simulink model "rotary_pendulum"  (R2022a)
settings: Solver=VariableStepAuto  StartTime=0.0  StopTime=2.5  RelTol=1e-3
values from neighbouring files (symbols this model uses):
  A = [0 0 1 0 ... (first row only)    [main.m]
  A_CL = A-B*K    [main.m]
  B = [0 ... (first row only)    [main.m]
  C = [1 0 0 0 ... (first row only)    [main.m]
  D = [0 ... (first row only)    [main.m]
  K = lqr(sys_ss, Q, R)    [main.m]
settings Model: Creator=punk  LastModifiedBy=punk

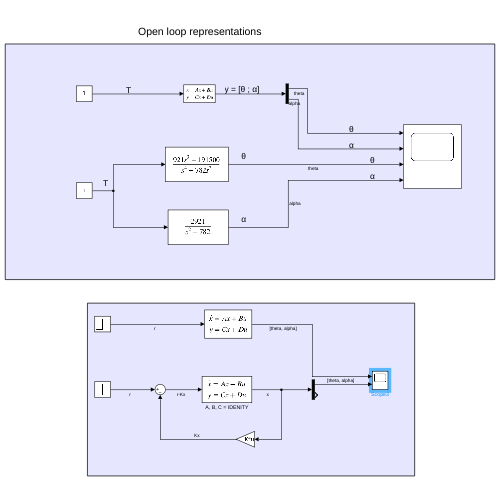
[thumbnail: Simulink's stored preview of the top-level diagram]
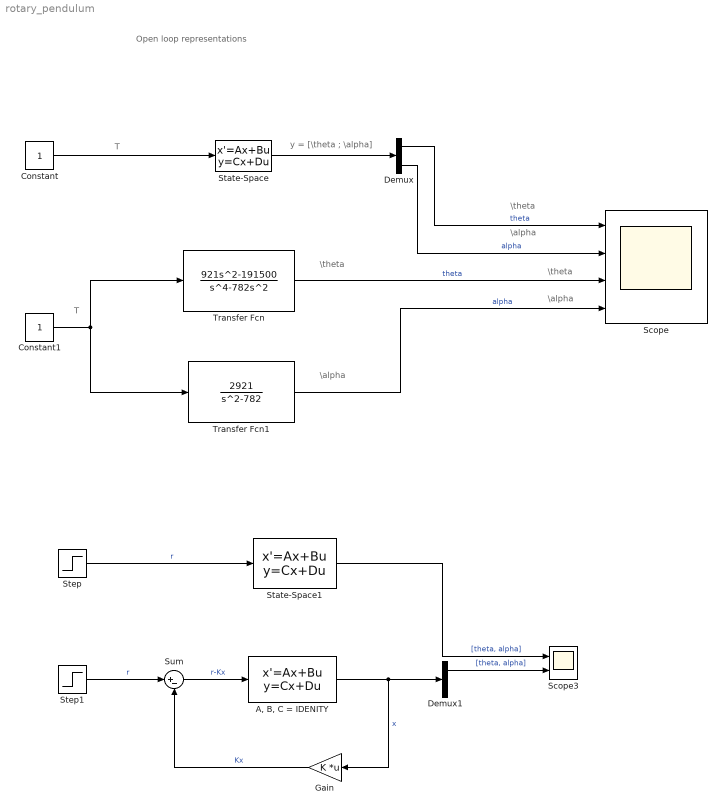
== system rotary_pendulum ==
  note: y = [\theta ; \alpha]
  note: T
  note: \alpha
  note: \theta
  note: Open loop representations
  note: T
  note: \theta
  note: \alpha
  note: \theta
  note: \alpha
  "A, B, C = IDENITY" : StateSpace  A=A  B=B  C=eye(4)  D=[0;0;0;0]  InitialCondition=0
  Constant : Constant
  Constant1 : Constant
  Demux : Demux  Outputs=2
  Demux1 : Demux  Outputs=2
  Gain : Gain  Gain=K  Multiplication=Matrix(K*u)
  Scope : Scope  NumInputPorts=4
  Scope3 : Scope  NumInputPorts=2
  State-Space : StateSpace  A=A  B=B  C=C  D=D  InitialCondition=0
  State-Space1 : StateSpace  A=A_CL  B=B  C=C  D=D  InitialCondition=0
  Step : Step  Time=0  SampleTime=0
  Step1 : Step  Time=0  SampleTime=0
  Sum : Sum  Inputs=|+-
  Transfer Fcn : TransferFcn  Numerator=[921 0 -191500]  Denominator=[1 0 -782 0 0]
  Transfer Fcn1 : TransferFcn  Numerator=[2921]  Denominator=[1 0 -782]
  wires:
  Constant/1 -> State-Space/1
  State-Space/1 -> Demux/1
  Transfer Fcn/1 -> Scope/3  "theta"
  Transfer Fcn1/1 -> Scope/4  "alpha"
  Constant1/1 -> Transfer Fcn1/1, Transfer Fcn/1
  Demux/1 -> Scope/1  "theta"
  Demux/2 -> Scope/2  "alpha"
  Step/1 -> State-Space1/1  "r"
  State-Space1/1 -> Scope3/1  "[theta, alpha]"
  Sum/1 -> "A, B, C = IDENITY"/1  "r-Kx"
  "A, B, C = IDENITY"/1 -> Demux1/1, Gain/1  "x"
  Gain/1 -> Sum/2  "Kx"
  Step1/1 -> Sum/1  "r"
  Demux1/1 -> Scope3/2  "[theta, alpha]"
